simulink model "practical_class_3_1b_simulink"  (R2023b)
settings: Solver=VariableStepAuto  StartTime=0.0  StopTime=9  MaxStep=1e-3  MinStep=1e-9  RelTol=1e-9
undefined symbols (not defined in the file): A, B, C, D
settings Model: Creator=klysm  LastModifiedBy=klysm
settings SolverCC: InitialStep=1e-9

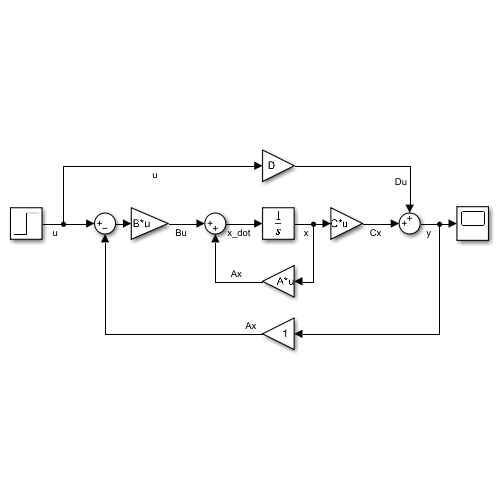
[thumbnail: Simulink's stored preview of the top-level diagram]
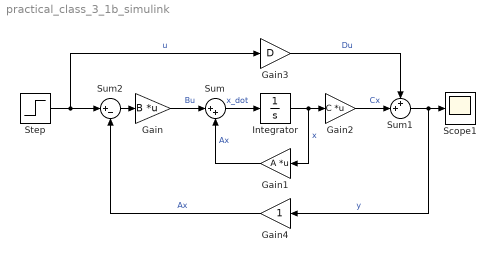
== system practical_class_3_1b_simulink ==
  Gain : Gain  Gain=B  Multiplication=Matrix(K*u)
  Gain1 : Gain  Gain=A  Multiplication=Matrix(K*u)
  Gain2 : Gain  Gain=C  Multiplication=Matrix(K*u)
  Gain3 : Gain  Gain=D
  Gain4 : Gain
  Integrator : Integrator
  Scope1 : Scope
  Step : Step  Time=0  SampleTime=0
  Sum : Sum  Inputs=|++
  Sum1 : Sum  Inputs=++|
  Sum2 : Sum  Inputs=|+-
  wires:
  Step/1 -> Sum2/1, Gain3/1  "u"
  Gain/1 -> Sum/1  "Bu"
  Sum/1 -> Integrator/1  "x_dot"
  Integrator/1 -> Gain1/1, Gain2/1  "x"
  Gain3/1 -> Sum1/1  "Du"
  Gain2/1 -> Sum1/2  "Cx"
  Gain1/1 -> Sum/2  "Ax"
  Sum1/1 -> Gain4/1, Scope1/1  "y"
  Sum2/1 -> Gain/1
  Gain4/1 -> Sum2/2  "Ax"
